simulink model "Askhsh_13c"  (R2018b)
settings: Solver=VariableStepAuto  StartTime=0.0  StopTime=20  RelTol=1e-3
libraries: simulink x4
settings Model: Creator=Argy  LastModifiedBy=Argy
settings DataIOCC: Refine=10

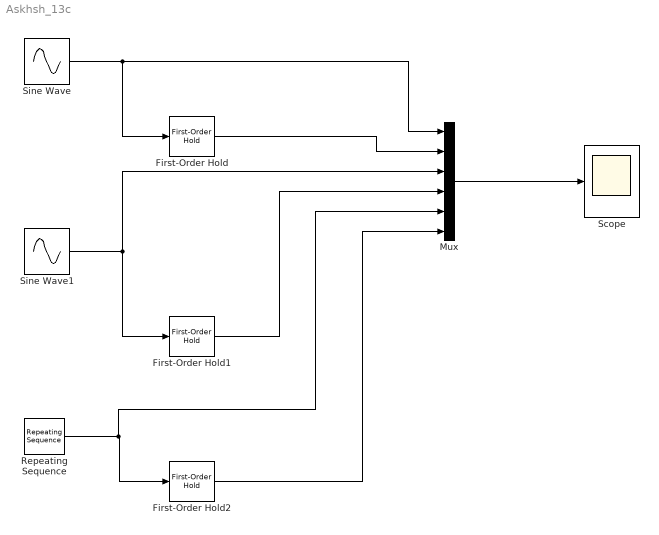
== system Askhsh_13c ==
  First-Order Hold : simulink/Discrete/First-Order Hold  DisableCoverage=on  Ts=0.1
      settings: SourceProductName=Simulink  SourceProductBaseCode=SL
  First-Order Hold1 : simulink/Discrete/First-Order Hold  DisableCoverage=on  Ts=0.1
      settings: SourceProductName=Simulink  SourceProductBaseCode=SL
  First-Order Hold2 : simulink/Discrete/First-Order Hold  DisableCoverage=on  Ts=0.1
      settings: SourceProductName=Simulink  SourceProductBaseCode=SL
  Mux : Mux  Inputs=6
  Repeating Sequence : simulink/Sources/Repeating Sequence  rep_seq_t=[0 2]  rep_seq_y=[-2 2]
  Scope : Scope
  Sine Wave : Sin  Amplitude=4  Frequency=10  SampleTime=0
  Sine Wave1 : Sin  Amplitude=2  Frequency=5  SampleTime=0
  wires:
  First-Order Hold/1 -> Mux/2
  Mux/1 -> Scope/1
  Sine Wave/1 -> First-Order Hold/1, Mux/1
  Sine Wave1/1 -> Mux/3, First-Order Hold1/1
  First-Order Hold1/1 -> Mux/4
  Repeating Sequence/1 -> Mux/5, First-Order Hold2/1
  First-Order Hold2/1 -> Mux/6
